simulink model "husky_sim_yichu_MPC_test"  (R2019b)
settings: Solver=ode4  StartTime=0.0  StopTime=5  FixedStep=Ts  MaxStep=0.001  RelTol=1e-3
InitFcn:
  | init_model;
values from neighbouring files (symbols this model uses):
  desired_input = [0,0,0,0,0,0,0,0,0,0,0,0]    [control_params_init.m]
  m = getfield(leg,'mass')    [dynamic_test.m]    (also in pen_init.m = link2.mass; test.mat = 2.2337)
  q_BL_K0 = initial_angle(12)    [func_params_ext.m]
  q_BR_K0 = initial_angle(9)    [func_params_ext.m]
  q_FL_K0 = initial_angle(6)    [func_params_ext.m]
  q_FR_K0 = initial_angle(3)    [func_params_ext.m]
undefined symbols (not defined in the file or in its folder): body, femur_left, femur_right, hip_left, hip_right, hipf_ctrl, hips_ctrl, knee_ctrl, link_left, link_right, tarsus_left, tarsus_right, tibia_left, tibia_right, X, Y, Z
libraries: sm_lib x247, nesl_utility x86, simulink x36, Contact_Forces_Lib x20
(part 1 of 9)
settings Model: PauseTimes=0.4  NumberOfSteps=10  SnapshotBufferSize=100  SnapshotInterval=20  Creator=Yang  LastModifiedBy=yichu
settings SolverCC: AlgebraicLoopSolver=LineSearch  SolverResetMethod=Robust
settings SFSimCC: CustomCodeUndefinedFunction=UseInterfaceOnly
settings RTWCC: Description=Simulink Desktop Real-Time  SystemTargetFile=sldrt.tlc  TemplateMakefile=sldrt.tmf  RTWCompilerOptimization=on
settings CodeAppCC: MaxIdLength=95
settings SimulinkDesktopRealTimeCC: TargetPreCompLibLocation=D:\Program Files\MATLAB\toolbox\sldrt\lib\win64  PreserveStateflowLocalDataDimensions=off
settings DiagnosticsConfigSet: SimMechanicsRigidlyBoundBlock=warning

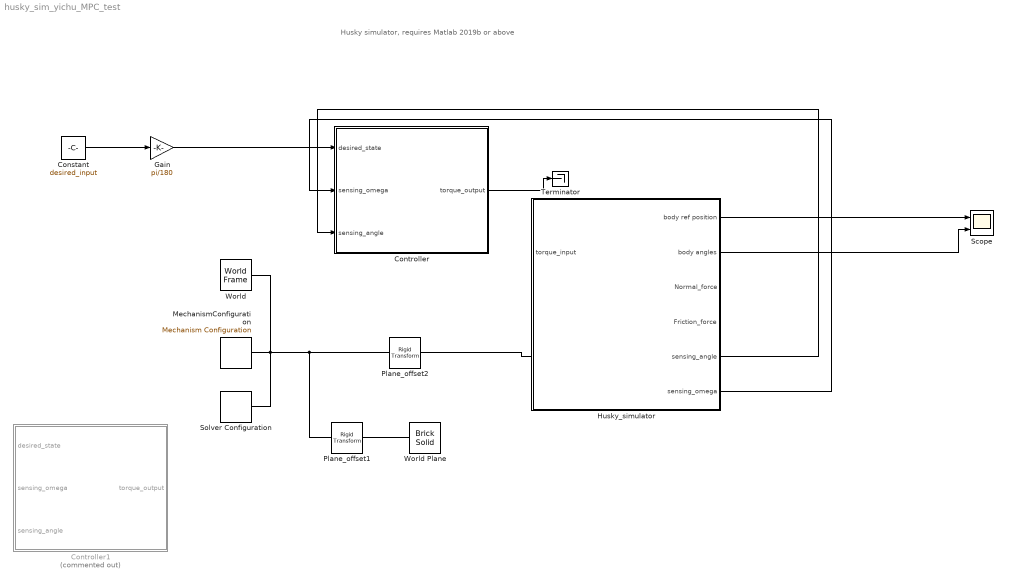
== system husky_sim_yichu_MPC_test ==
  note: Husky simulator, requires Matlab 2019b or above
  Constant : Constant  Value=desired_input
  Controller : Subsystem
  Controller1 : Subsystem  Commented=on
  Gain : Gain  Gain=pi/180
  Husky_simulator : Subsystem
  MechanismConfiguration : sm_lib/Utilities/Mechanism Configuration  UniformGravity=Constant  GravityVector=[0 0 -9.80665]  GravityUnits=m/s^2  LinearizationDelta=0.001
  Plane_offset1 : sm_lib/Frames and Transforms/Rigid Transform  TranslationMethod=Cartesian  TranslationStandardOffset=0  TranslationLengthUnit=m  TranslationStandardAxis=+Z  TranslationCartesianOffset=[0, 0, 0]  TranslationROffset=0  TranslationROffsetUnits=m  TranslationZOffset=0  TranslationZOffsetUnits=m  TranslationThetaOffset=0  TranslationThetaOffsetUnits=deg  RotationMethod=RotationSequence  RotationAngleUnits=deg  RotationStandardAxis=+Z  RotationAngle=0.0  RotationArbitraryAxis=[0 0 1]  FollAlignAxisA=+X  BaseAlignAxisA=+Y  FollAlignAxisB=+Y  BaseAlignAxisB=+Z  RotationSequenceAxes=BaseAxes  RotationSequence=XYZ  RotationSequenceAngles=[0, 0, 0]  RotationSequenceAnglesUnits=rad  RotationMatrix=[1 0 0; 0 1 0; 0 0 1]
  Plane_offset2 : sm_lib/Frames and Transforms/Rigid Transform  TranslationMethod=Cartesian  TranslationStandardOffset=0  TranslationLengthUnit=m  TranslationStandardAxis=+Z  TranslationCartesianOffset=[0, 0, 0]  TranslationROffset=0  TranslationROffsetUnits=m  TranslationZOffset=0  TranslationZOffsetUnits=m  TranslationThetaOffset=0  TranslationThetaOffsetUnits=deg  RotationMethod=StandardAxis  RotationAngleUnits=deg  RotationStandardAxis=+Z  RotationAngle=-90  RotationArbitraryAxis=[0 0 1]  FollAlignAxisA=+X  BaseAlignAxisA=+Y  FollAlignAxisB=+Y  BaseAlignAxisB=+Z  RotationSequenceAxes=BaseAxes  RotationSequence=XYZ  RotationSequenceAngles=[0, 0, 0]  RotationSequenceAnglesUnits=rad  RotationMatrix=[1 0 0; 0 1 0; 0 0 1]
  Scope : Scope  NumInputPorts=2
  Solver Configuration : nesl_utility/Solver Configuration  PhysicalDomain=network_engine_domain  SubClassName=solver  LeftPortType=input  RightPortType=generic  Tones=[]  Harmonics=[]  SimulateNoise=off  Profile=off  UseLocalSampling=off  EnableSwitchedLinearOptims=on  FrequencyDomain=off  UseCCode=off  RelTol=0.001  AbsTol=1e-06  MinStep=1e-09  ToWorkspace=off  RevertToSquareIcSolve=off  NumHomotopyIterations=100  PhasorMode=off  PhasorModeNumHarmonics=1  DoDC=off  ResidualTolerance=1e-09  UseLocalSolver=off  LocalSolverChoice=NE_BACKWARD_EULER_ADVANCER  LocalSolverSampleTime=0.001  DoFixedCost=off  MaxNonlinIter=3  MaxModeIter=2  LinearAlgebra=auto  EquationFormulation=NE_TIME_EF  DelaysMemoryBudget=1024  AutomaticFiltering=on  FilteringTimeConstant=0.001  PartitionStorageMethod=AS_NEEDED  PartitionMemoryBudget=1024  PartitionMethod=ROBUST
  Terminator : Terminator
  World : sm_lib/Frames and Transforms/World Frame
  "World Plane " : sm_lib/Body Elements/Brick Solid  GraphicAmbientColor=[0.15 0.15 0.15 1.0]  BasedOnType=Density  BrickDimensions=[5 5 0.02]  BrickDimensionUnits=m  CenterOfMass=[0 0 0]  CenterOfMassUnits=m  GraphicDiffuseColor=[0.5 0.5 0.5]  Density=1000  DensityUnits=kg/m^3  DoExposeReferenceFrame=on  GraphicEmissiveColor=[0.0 0.0 0.0 1.0]  ExportEntireGeometry=off  SerializedFrames=<Frames/>  MarkerShape=Sphere  MarkerSize=10  GraphicType=FromGeometry  InertiaType=CalculateFromGeometry  Mass=1  MassUnits=kg  MomentsOfInertia=[1 1 1]  MomentsOfInertiaUnits=kg*m^2  GraphicOpacity=1.0  ProductsOfInertia=[0 0 0]  ProductsOfInertiaUnits=kg*m^2  GraphicShininess=75  GraphicSpecularColor=[0.5 0.5 0.5 1.0]  GraphicVisPropType=SimpleVisualProperties
  wires:
  Controller/1(torque_output) -> Terminator/1
  Husky_simulator/5(sensing_angle) -> Controller/3(sensing_angle)
  Husky_simulator/6(sensing_omega) -> Controller/2(sensing_omega)
  Constant/1 -> Gain/1
  Gain/1 -> Controller/1("desired_state ")
  Husky_simulator/2(body angles) -> Scope/2
  Husky_simulator/1(body ref position) -> Scope/1
  connections:
  Plane_offset2/RConn1 -- Husky_simulator/LConn1
  Plane_offset1/RConn1 -- "World Plane "/RConn1
  Plane_offset1/LConn1 -- Plane_offset2/LConn1 -- Solver Configuration/RConn1 -- World/RConn1 -- MechanismConfiguration/RConn1

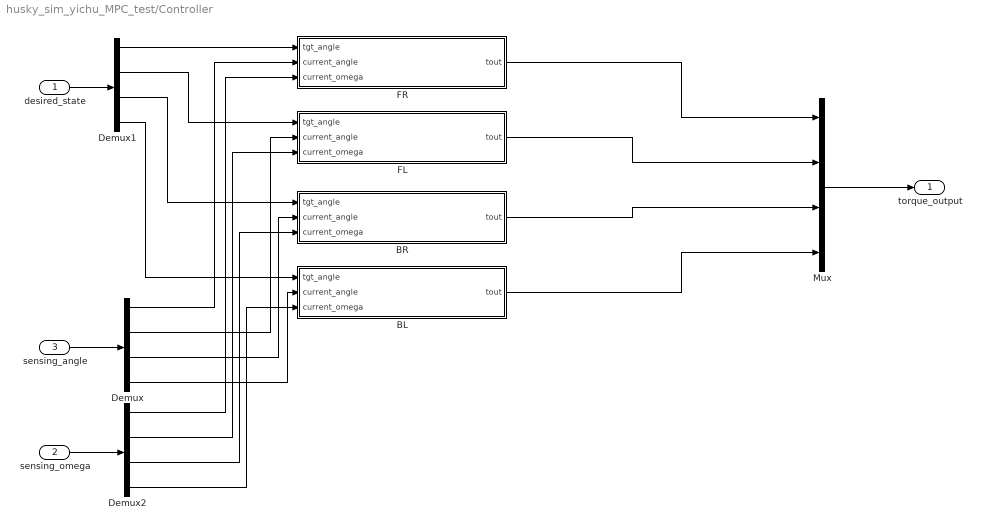
== system husky_sim_yichu_MPC_test/Controller ==
  "desired_state " : Inport
  sensing_omega : Inport  Port=2
  sensing_angle : Inport  Port=3
  BL : Subsystem
  BR : Subsystem
  Demux : Demux
  Demux1 : Demux
  Demux2 : Demux
  FL : Subsystem
  "FR " : Subsystem
  Mux : Mux
  torque_output : Outport
  wires:
  sensing_angle/1 -> Demux/1
  "desired_state "/1 -> Demux1/1
  Demux/1 -> "FR "/2("current_angle ")
  Demux/2 -> FL/2("current_angle ")
  Demux/3 -> BR/2("current_angle ")
  Demux/4 -> BL/2("current_angle ")
  Demux1/1 -> "FR "/1(tgt_angle)
  Demux1/2 -> FL/1(tgt_angle)
  Demux1/3 -> BR/1(tgt_angle)
  Demux1/4 -> BL/1(tgt_angle)
  Demux2/4 -> BL/3(current_omega)
  sensing_omega/1 -> Demux2/1
  Demux2/1 -> "FR "/3(current_omega)
  Demux2/3 -> BR/3(current_omega)
  Demux2/2 -> FL/3(current_omega)
  "FR "/1("tout ") -> Mux/1
  FL/1("tout ") -> Mux/2
  BR/1("tout ") -> Mux/3
  BL/1("tout ") -> Mux/4
  Mux/1 -> torque_output/1

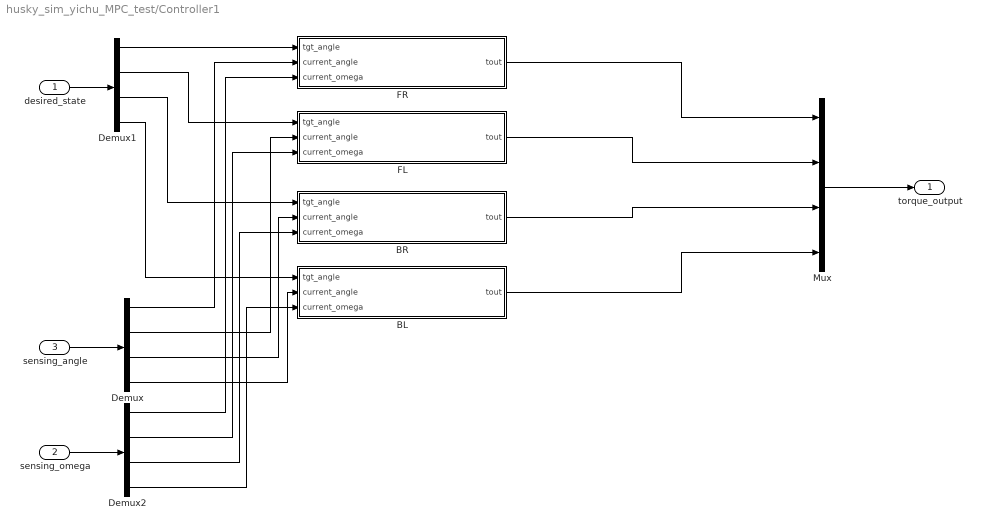
== system husky_sim_yichu_MPC_test/Controller1 ==
  "desired_state " : Inport
  sensing_omega : Inport  Port=2
  sensing_angle : Inport  Port=3
  BL : Subsystem
  BR : Subsystem
  Demux : Demux
  Demux1 : Demux
  Demux2 : Demux
  FL : Subsystem
  "FR " : Subsystem
  Mux : Mux
  torque_output : Outport
  wires:
  sensing_angle/1 -> Demux/1
  "desired_state "/1 -> Demux1/1
  Demux/1 -> "FR "/2("current_angle ")
  Demux/2 -> FL/2("current_angle ")
  Demux/3 -> BR/2("current_angle ")
  Demux/4 -> BL/2("current_angle ")
  Demux1/1 -> "FR "/1(tgt_angle)
  Demux1/2 -> FL/1(tgt_angle)
  Demux1/3 -> BR/1(tgt_angle)
  Demux1/4 -> BL/1(tgt_angle)
  Demux2/4 -> BL/3(current_omega)
  sensing_omega/1 -> Demux2/1
  Demux2/1 -> "FR "/3(current_omega)
  Demux2/3 -> BR/3(current_omega)
  Demux2/2 -> FL/3(current_omega)
  "FR "/1("tout ") -> Mux/1
  FL/1("tout ") -> Mux/2
  BR/1("tout ") -> Mux/3
  BL/1("tout ") -> Mux/4
  Mux/1 -> torque_output/1

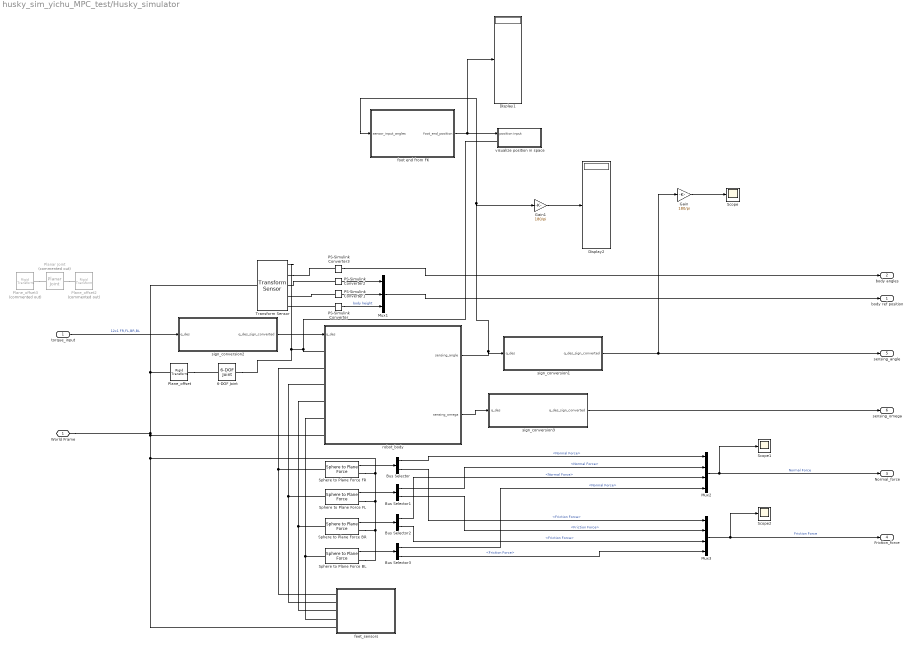
== system husky_sim_yichu_MPC_test/Husky_simulator ==
  "torque_input " : Inport
  6-DOF Joint : sm_lib/Joints/6-DOF Joint  JointMode=Normal  SenseConstraintForce=off  SenseConstraintForceX=off  SenseConstraintForceY=off  SenseConstraintForceZ=off  SenseConstraintTorque=off  SenseConstraintTorqueX=off  SenseConstraintTorqueY=off  SenseConstraintTorqueZ=off  SenseTotalForce=off  SenseTotalForceX=off  SenseTotalForceY=off  SenseTotalForceZ=off  SenseTotalTorque=off  SenseTotalTorqueX=off  SenseTotalTorqueY=off  SenseTotalTorqueZ=off  CompositeWrenchDir=FollowerOnBase  CompositeWrenchFrame=BaseFrame  PxEquilibriumPosition=0  PxEquilibriumPositionUnits=m  PxSpringStiffness=0  PxSpringStiffnessUnits=N/m  PxDampingCoefficient=0  PxDampingCoefficientUnits=N/(m/s)  PxTorqueActuationMode=NoTorque  PxMotionActuationMode=ComputedMotion  PxSensePosition=off  PxSenseVelocity=off  PxSenseAcceleration=off  PxSenseTorqueForce=off  PxSenseLowerLimitTorqueForce=off  PxSenseUpperLimitTorqueForce=off  PxLowerLimitSpecify=off  PxLowerLimitBound=-1  PxLowerLimitBoundUnits=m  PxLowerLimitStiffness=1e6  PxLowerLimitStiffnessUnits=N/m  PxLowerLimitDamping=1e3  PxLowerLimitDampingUnits=N/(m/s)  PxLowerLimitTransitionRegionWidth=1e-4  PxLowerLimitTransitionRegionWidthUnits=m  PxUpperLimitSpecify=off  PxUpperLimitBound=1  PxUpperLimitBoundUnits=m  PxUpperLimitStiffness=1e6  PxUpperLimitStiffnessUnits=N/m  PxUpperLimitDamping=1e3  PxUpperLimitDampingUnits=N/(m/s)  PxUpperLimitTransitionRegionWidth=1e-4  PxUpperLimitTransitionRegionWidthUnits=m  PxPositionTargetSpecify=off  PxPositionTargetPriority=High  PxPositionTargetValue=0  PxPositionTargetValueUnits=m  PxVelocityTargetSpecify=off  PxVelocityTargetPriority=High  PxVelocityTargetValue=0  PxVelocityTargetValueUnits=m/s  PyEquilibriumPosition=0  PyEquilibriumPositionUnits=m  PySpringStiffness=0  PySpringStiffnessUnits=N/m  PyDampingCoefficient=0  PyDampingCoefficientUnits=N/(m/s)  PyTorqueActuationMode=NoTorque  PyMotionActuationMode=ComputedMotion  PySensePosition=off  PySenseVelocity=off  PySenseAcceleration=off  PySenseTorqueForce=off  PySenseLowerLimitTorqueForce=off  PySenseUpperLimitTorqueForce=off  PyLowerLimitSpecify=off  PyLowerLimitBound=-1  PyLowerLimitBoundUnits=m  PyLowerLimitStiffness=1e6  PyLowerLimitStiffnessUnits=N/m  PyLowerLimitDamping=1e3  PyLowerLimitDampingUnits=N/(m/s)  PyLowerLimitTransitionRegionWidth=1e-4  PyLowerLimitTransitionRegionWidthUnits=m  PyUpperLimitSpecify=off  PyUpperLimitBound=1  PyUpperLimitBoundUnits=m  PyUpperLimitStiffness=1e6  PyUpperLimitStiffnessUnits=N/m  PyUpperLimitDamping=1e3  PyUpperLimitDampingUnits=N/(m/s)  PyUpperLimitTransitionRegionWidth=1e-4  PyUpperLimitTransitionRegionWidthUnits=m  PyPositionTargetSpecify=off  PyPositionTargetPriority=High  PyPositionTargetValue=0  PyPositionTargetValueUnits=m  PyVelocityTargetSpecify=off  PyVelocityTargetPriority=High  PyVelocityTargetValue=0  PyVelocityTargetValueUnits=m/s  PzEquilibriumPosition=0  PzEquilibriumPositionUnits=m  PzSpringStiffness=0  PzSpringStiffnessUnits=N/m  PzDampingCoefficient=0  PzDampingCoefficientUnits=N/(m/s)  PzTorqueActuationMode=NoTorque  PzMotionActuationMode=ComputedMotion  PzSensePosition=off  PzSenseVelocity=off  PzSenseAcceleration=off  PzSenseTorqueForce=off  PzSenseLowerLimitTorqueForce=off  PzSenseUpperLimitTorqueForce=off  PzLowerLimitSpecify=off  PzLowerLimitBound=-1  PzLowerLimitBoundUnits=m  PzLowerLimitStiffness=1e6  PzLowerLimitStiffnessUnits=N/m  PzLowerLimitDamping=1e3  PzLowerLimitDampingUnits=N/(m/s)  PzLowerLimitTransitionRegionWidth=1e-4  PzLowerLimitTransitionRegionWidthUnits=m  PzUpperLimitSpecify=off  PzUpperLimitBound=1  PzUpperLimitBoundUnits=m  PzUpperLimitStiffness=1e6  PzUpperLimitStiffnessUnits=N/m  PzUpperLimitDamping=1e3  PzUpperLimitDampingUnits=N/(m/s)  PzUpperLimitTransitionRegionWidth=1e-4  PzUpperLimitTransitionRegionWidthUnits=m  PzPositionTargetSpecify=off  PzPositionTargetPriority=High  PzPositionTargetValue=0  PzPositionTargetValueUnits=m  PzVelocityTargetSpecify=off  PzVelocityTargetPriority=High  PzVelocityTargetValue=0  PzVelocityTargetValueUnits=m/s  SphDefPosRotationMethod=None  SphDefPosRotationAngleUnits=deg  SphDefPosRotationStandardAxis=+Z  SphDefPosRotationAngle=0.0  SphDefPosRotationArbitraryAxis=[0 0 1]  SphDefPosFollAlignAxisA=+X  SphDefPosBaseAlignAxisA=+Y  SphDefPosFollAlignAxisB=+Y  SphDefPosBaseAlignAxisB=+Z  SphDefPosRotationSequenceAxes=FollowerAxes  SphDefPosRotationSequence=XYX  SphDefPosRotationSequenceAngles=[0 0 0]  SphDefPosRotationSequenceAnglesUnits=deg  SphDefPosRotationMatrix=[1 0 0; 0 1 0; 0 0 1]  SphEqPosRotationMethod=None  SphEqPosRotationAngleUnits=deg  SphEqPosRotationStandardAxis=+Z  SphEqPosRotationAngle=0.0  SphEqPosRotationArbitraryAxis=[0 0 1]  SphEqPosFollAlignAxisA=+X  SphEqPosBaseAlignAxisA=+Y  SphEqPosFollAlignAxisB=+Y  SphEqPosBaseAlignAxisB=+Z  SphEqPosRotationSequenceAxes=FollowerAxes  SphEqPosRotationSequence=XYX  SphEqPosRotationSequenceAngles=[0 0 0]  SphEqPosRotationSequenceAnglesUnits=deg  SphEqPosRotationMatrix=[1 0 0; 0 1 0; 0 0 1]  SphSpringStiffness=0  SphSpringStiffnessUnits=N*m/deg  SphDampingCoefficient=0  SphDampingCoefficientUnits=N*m/(deg/s)  SphActuateTorqueX=off  SphActuateTorqueY=off  SphActuateTorqueZ=off  SphActuateTorque=off  SphTorqueActuationMode=NoTorque  SphMotionActuationMode=ComputedMotion  SphActuationFrame=BaseFrame  SphSensePosition=off  SphSenseVelocityX=off  SphSenseVelocityY=off  SphSenseVelocityZ=off  SphSenseVelocity=off  SphSenseAccelerationX=off  SphSenseAccelerationY=off  SphSenseAccelerationZ=off  SphSenseAcceleration=off  SphSenseTorqueX=off  SphSenseTorqueY=off  SphSenseTorqueZ=off  SphSenseTorqueForce=off  SphSenseLowerLimitTorqueMag=off  SphSenseUpperLimitTorqueMag=off  SphSensingFrame=BaseFrame  SphLowerLimitSpecify=off  SphLowerLimitBound=15  SphLowerLimitBoundUnits=deg  SphLowerLimitStiffness=1e4  SphLowerLimitStiffnessUnits=N*m/deg  SphLowerLimitDamping=10  SphLowerLimitDampingUnits=N*m/(deg/s)  SphLowerLimitTransitionRegionWidth=0.1  SphLowerLimitTransitionRegionWidthUnits=deg  SphUpperLimitSpecify=off  SphUpperLimitBound=45  SphUpperLimitBoundUnits=deg  SphUpperLimitStiffness=1e4  SphUpperLimitStiffnessUnits=N*m/deg  SphUpperLimitDamping=10  SphUpperLimitDampingUnits=N*m/(deg/s)  SphUpperLimitTransitionRegionWidth=0.1  SphUpperLimitTransitionRegionWidthUnits=deg  SphPositionTargetRotationMethod=None  SphPositionTargetRotationAngleUnits=deg  SphPositionTargetRotationStandardAxis=+Z  SphPositionTargetRotationAngle=0.0  SphPositionTargetRotationArbitraryAxis=[0 0 1]  SphPositionTargetFollAlignAxisA=+X  SphPositionTargetBaseAlignAxisA=+Y  SphPositionTargetFollAlignAxisB=+Y  SphPositionTargetBaseAlignAxisB=+Z  SphPositionTargetRotationSequenceAxes=FollowerAxes  SphPositionTargetRotationSequence=XYX  SphPositionTargetRotationSequenceAngles=[0 0 0]  SphPositionTargetRotationSequenceAnglesUnits=deg  SphPositionTargetRotationMatrix=[1 0 0; 0 1 0; 0 0 1]  SphPositionTargetSpecify=off  SphPositionTargetPriority=High  SphVelocityTargetValue=[0 0 0]  SphVelocityTargetValueUnits=deg/s  SphVelocityTargetSpecify=off  SphVelocityTargetPriority=High  SphVelocityTargetInFollowerFrame=on
  Bus Selector{,1..3} (4 alike) : BusSelector  OutputSignals=Normal Force,Friction Force
  Display1 : Display
  Display2 : Display
  Gain : Gain  Gain=180/pi
  Gain1 : Gain  Gain=180/pi
  Mux1 : Mux  Inputs=3
  Mux2 : Mux
  Mux3 : Mux
  PS-Simulink Converter{,1..3} (4 alike) : nesl_utility/PS-Simulink Converter  PhysicalDomain=network_engine_domain  SubClassName=ps_output  LeftPortType=input  RightPortType=output  PseudoPeriodic=off  Frequencies=[]  Unit=inherit  AffineConversion=off
  Planar Joint : sm_lib/Joints/Planar Joint  Commented=on  JointMode=Normal  SenseConstraintForce=off  SenseConstraintForceX=off  SenseConstraintForceY=off  SenseConstraintForceZ=off  SenseConstraintTorque=off  SenseConstraintTorqueX=off  SenseConstraintTorqueY=off  SenseConstraintTorqueZ=off  SenseTotalForce=off  SenseTotalForceX=off  SenseTotalForceY=off  SenseTotalForceZ=off  SenseTotalTorque=off  SenseTotalTorqueX=off  SenseTotalTorqueY=off  SenseTotalTorqueZ=off  CompositeWrenchDir=FollowerOnBase  CompositeWrenchFrame=BaseFrame  PxEquilibriumPosition=0  PxEquilibriumPositionUnits=m  PxSpringStiffness=0  PxSpringStiffnessUnits=N/m  PxDampingCoefficient=0  PxDampingCoefficientUnits=N/(m/s)  PxTorqueActuationMode=NoTorque  PxMotionActuationMode=ComputedMotion  PxSensePosition=off  PxSenseVelocity=off  PxSenseAcceleration=off  PxSenseTorqueForce=off  PxSenseLowerLimitTorqueForce=off  PxSenseUpperLimitTorqueForce=off  PxLowerLimitSpecify=off  PxLowerLimitBound=-1  PxLowerLimitBoundUnits=m  PxLowerLimitStiffness=1e6  PxLowerLimitStiffnessUnits=N/m  PxLowerLimitDamping=1e3  PxLowerLimitDampingUnits=N/(m/s)  PxLowerLimitTransitionRegionWidth=1e-4  PxLowerLimitTransitionRegionWidthUnits=m  PxUpperLimitSpecify=off  PxUpperLimitBound=1  PxUpperLimitBoundUnits=m  PxUpperLimitStiffness=1e6  PxUpperLimitStiffnessUnits=N/m  PxUpperLimitDamping=1e3  PxUpperLimitDampingUnits=N/(m/s)  PxUpperLimitTransitionRegionWidth=1e-4  PxUpperLimitTransitionRegionWidthUnits=m  PxPositionTargetSpecify=off  PxPositionTargetPriority=High  PxPositionTargetValue=0  PxPositionTargetValueUnits=m  PxVelocityTargetSpecify=off  PxVelocityTargetPriority=High  PxVelocityTargetValue=0  PxVelocityTargetValueUnits=m/s  PyEquilibriumPosition=0  PyEquilibriumPositionUnits=m  PySpringStiffness=0  PySpringStiffnessUnits=N/m  PyDampingCoefficient=0  PyDampingCoefficientUnits=N/(m/s)  PyTorqueActuationMode=NoTorque  PyMotionActuationMode=ComputedMotion  PySensePosition=off  PySenseVelocity=off  PySenseAcceleration=off  PySenseTorqueForce=off  PySenseLowerLimitTorqueForce=off  PySenseUpperLimitTorqueForce=off  PyLowerLimitSpecify=off  PyLowerLimitBound=-1  PyLowerLimitBoundUnits=m  PyLowerLimitStiffness=1e6  PyLowerLimitStiffnessUnits=N/m  PyLowerLimitDamping=1e3  PyLowerLimitDampingUnits=N/(m/s)  PyLowerLimitTransitionRegionWidth=1e-4  PyLowerLimitTransitionRegionWidthUnits=m  PyUpperLimitSpecify=off  PyUpperLimitBound=1  PyUpperLimitBoundUnits=m  PyUpperLimitStiffness=1e6  PyUpperLimitStiffnessUnits=N/m  PyUpperLimitDamping=1e3  PyUpperLimitDampingUnits=N/(m/s)  PyUpperLimitTransitionRegionWidth=1e-4  PyUpperLimitTransitionRegionWidthUnits=m  PyPositionTargetSpecify=off  PyPositionTargetPriority=High  PyPositionTargetValue=0  PyPositionTargetValueUnits=m  PyVelocityTargetSpecify=off  PyVelocityTargetPriority=High  PyVelocityTargetValue=0  PyVelocityTargetValueUnits=m/s  RzEquilibriumPosition=0  RzEquilibriumPositionUnits=deg  RzSpringStiffness=0  RzSpringStiffnessUnits=N*m/deg  RzDampingCoefficient=0  RzDampingCoefficientUnits=N*m/(deg/s)  RzTorqueActuationMode=NoTorque  RzMotionActuationMode=ComputedMotion  RzSensePosition=off  RzSenseVelocity=off  RzSenseAcceleration=off  RzSenseTorqueForce=off  RzSenseLowerLimitTorqueForce=off  RzSenseUpperLimitTorqueForce=off  RzLowerLimitSpecify=off  RzLowerLimitBound=-90  RzLowerLimitBoundUnits=deg  RzLowerLimitStiffness=1e4  RzLowerLimitStiffnessUnits=N*m/deg  RzLowerLimitDamping=10  RzLowerLimitDampingUnits=N*m/(deg/s)  RzLowerLimitTransitionRegionWidth=0.1  RzLowerLimitTransitionRegionWidthUnits=deg  RzUpperLimitSpecify=off  RzUpperLimitBound=90  RzUpperLimitBoundUnits=deg  RzUpperLimitStiffness=1e4  RzUpperLimitStiffnessUnits=N*m/deg  RzUpperLimitDamping=10  RzUpperLimitDampingUnits=N*m/(deg/s)  RzUpperLimitTransitionRegionWidth=0.1  RzUpperLimitTransitionRegionWidthUnits=deg  RzPositionTargetSpecify=off  RzPositionTargetPriority=High  RzPositionTargetValue=0  RzPositionTargetValueUnits=deg  RzVelocityTargetSpecify=off  RzVelocityTargetPriority=High  RzVelocityTargetValue=0  RzVelocityTargetValueUnits=deg/s
  Plane_offset : sm_lib/Frames and Transforms/Rigid Transform  TranslationMethod=Cartesian  TranslationStandardOffset=0  TranslationLengthUnit=m  TranslationStandardAxis=+Z  TranslationCartesianOffset=p_b0  TranslationROffset=0  TranslationROffsetUnits=m  TranslationZOffset=0  TranslationZOffsetUnits=m  TranslationThetaOffset=0  TranslationThetaOffsetUnits=deg  RotationMethod=RotationSequence  RotationAngleUnits=deg  RotationStandardAxis=+Z  RotationAngle=0.0  RotationArbitraryAxis=[0 0 1]  FollAlignAxisA=+X  BaseAlignAxisA=+Y  FollAlignAxisB=+Y  BaseAlignAxisB=+Z  RotationSequenceAxes=BaseAxes  RotationSequence=XYZ  RotationSequenceAngles=[0, 0, 0]  RotationSequenceAnglesUnits=deg  RotationMatrix=[1 0 0; 0 1 0; 0 0 1]
  Plane_offset2 : sm_lib/Frames and Transforms/Rigid Transform  Commented=on  TranslationMethod=Cartesian  TranslationStandardOffset=0  TranslationLengthUnit=m  TranslationStandardAxis=+Z  TranslationCartesianOffset=[0, 0, 0]  TranslationROffset=0  TranslationROffsetUnits=m  TranslationZOffset=0  TranslationZOffsetUnits=m  TranslationThetaOffset=0  TranslationThetaOffsetUnits=deg  RotationMethod=RotationSequence  RotationAngleUnits=deg  RotationStandardAxis=+Z  RotationAngle=0.0  RotationArbitraryAxis=[0 0 1]  FollAlignAxisA=+X  BaseAlignAxisA=+Y  FollAlignAxisB=+Y  BaseAlignAxisB=+Z  RotationSequenceAxes=BaseAxes  RotationSequence=XYZ  RotationSequenceAngles=[-90, 0, 0]  RotationSequenceAnglesUnits=deg  RotationMatrix=[1 0 0; 0 1 0; 0 0 1]
  Plane_offset3 : sm_lib/Frames and Transforms/Rigid Transform  Commented=on  TranslationMethod=Cartesian  TranslationStandardOffset=0  TranslationLengthUnit=m  TranslationStandardAxis=+Z  TranslationCartesianOffset=[0, 0, 0]  TranslationROffset=0  TranslationROffsetUnits=m  TranslationZOffset=0  TranslationZOffsetUnits=m  TranslationThetaOffset=0  TranslationThetaOffsetUnits=deg  RotationMethod=RotationSequence  RotationAngleUnits=deg  RotationStandardAxis=+Z  RotationAngle=0.0  RotationArbitraryAxis=[0 0 1]  FollAlignAxisA=+X  BaseAlignAxisA=+Y  FollAlignAxisB=+Y  BaseAlignAxisB=+Z  RotationSequenceAxes=BaseAxes  RotationSequence=XYZ  RotationSequenceAngles=[90, 0, 0]  RotationSequenceAnglesUnits=deg  RotationMatrix=[1 0 0; 0 1 0; 0 0 1]
  Scope : Scope
  Scope1 : Scope
  Scope2 : Scope
  "Sphere to Plane Force BL " : Contact_Forces_Lib/3D/Sphere to Plane Force  sphere_rad=0.021  plane_lenx=5  plane_leny=5  plane_depth=0.01  force_law=Linear  k_contact=c_k  b_contact=c_b  pen_full_damp_F=1e-4  pen_exponent=1  custom_param_1=1  custom_param_2=1  friction_law=Stick-Slip Continuous  mu_kinetic=mu_k  mu_static=mu_s  v_thr=v_th  vis_on=off  vis_opc_en=0  vis_len_plaBz=0.001  vis_clr=[0.9 0.2 0.2]  vis_opc=0.7
  "Sphere to Plane Force BR " : Contact_Forces_Lib/3D/Sphere to Plane Force  sphere_rad=0.021  plane_lenx=5  plane_leny=5  plane_depth=0.01  force_law=Linear  k_contact=c_k  b_contact=c_b  pen_full_damp_F=1e-4  pen_exponent=1  custom_param_1=1  custom_param_2=1  friction_law=Stick-Slip Continuous  mu_kinetic=mu_k  mu_static=mu_s  v_thr=v_th  vis_on=off  vis_opc_en=0  vis_len_plaBz=0.001  vis_clr=[0.9 0.2 0.2]  vis_opc=0.7
  Sphere to Plane Force FL : Contact_Forces_Lib/3D/Sphere to Plane Force  sphere_rad=0.021  plane_lenx=5  plane_leny=5  plane_depth=0.01  force_law=Linear  k_contact=c_k  b_contact=c_b  pen_full_damp_F=1e-4  pen_exponent=1  custom_param_1=1  custom_param_2=1  friction_law=Stick-Slip Continuous  mu_kinetic=mu_k  mu_static=mu_s  v_thr=v_th  vis_on=off  vis_opc_en=0  vis_len_plaBz=0.001  vis_clr=[0.9 0.2 0.2]  vis_opc=0.7
  Sphere to Plane Force FR : Contact_Forces_Lib/3D/Sphere to Plane Force  sphere_rad=0.021  plane_lenx=5  plane_leny=5  plane_depth=0.01  force_law=Linear  k_contact=c_k  b_contact=c_b  pen_full_damp_F=1e-4  pen_exponent=1  custom_param_1=1  custom_param_2=1  friction_law=Stick-Slip Continuous  mu_kinetic=mu_k  mu_static=mu_s  v_thr=v_th  vis_on=off  vis_opc_en=0  vis_len_plaBz=0.001  vis_clr=[0.9 0.2 0.2]  vis_opc=0.7
  Transform Sensor : sm_lib/Frames and Transforms/Transform Sensor  MeasurementFrame=World  SenseAngle=off  SenseAxis=off  SenseAngle1=off  SenseAngle2=off  SenseAngle3=off  SenseQ=on  SenseR=off  SenseOmegaX=off  SenseOmegaY=off  SenseOmegaZ=off  SenseOmega1=off  SenseOmega2=off  SenseOmega3=off  SenseQDot=off  SenseRDot=off  SenseAlphaX=off  SenseAlphaY=off  SenseAlphaZ=off  SenseAlpha1=off  SenseAlpha2=off  SenseAlpha3=off  SenseQDDot=off  SenseRDDot=off  SenseX=on  SenseY=on  SenseZ=on  SenseRad=off  SenseAzim=off  SenseDist=off  SenseInc=off  SenseXDot=off  SenseYDot=off  SenseZDot=off  SenseRadDot=off  SenseAzimDot=off  SenseDistDot=off  SenseIncDot=off  SenseXDDot=off  SenseYDDot=off  SenseZDDot=off  SenseRadDDot=off  SenseAzimDDot=off  SenseDistDDot=off  SenseIncDDot=off
  feet_sensors : Subsystem
  "foot end from FK " : Subsystem
  robot_body : Subsystem
  sign_conversion1 : MATLAB Function  TreatAsAtomicUnit=on
  sign_conversion2 : MATLAB Function  TreatAsAtomicUnit=on
  sign_conversion3 : MATLAB Function  TreatAsAtomicUnit=on
  "visualize position in space " : Subsystem
  World Frame : PMIOPort  Side=Left
  body ref position : Outport
  body angles : Outport  Port=2
  Normal_force : Outport  Port=3
  Friction_force : Outport  Port=4
  sensing_angle : Outport  Port=5  VectorParamsAs1DForOutWhenUnconnected=off
  sensing_omega : Outport  Port=6  VectorParamsAs1DForOutWhenUnconnected=off
  wires:
  Sphere to Plane Force FR/1 -> Bus Selector/1
  Sphere to Plane Force FL/1 -> Bus Selector1/1
  "Sphere to Plane Force BR "/1 -> Bus Selector2/1
  "Sphere to Plane Force BL "/1 -> Bus Selector3/1
  PS-Simulink Converter/1 -> Mux1/3  "body height"
  PS-Simulink Converter2/1 -> Mux1/1
  PS-Simulink Converter1/1 -> Mux1/2
  Mux1/1 -> body ref position/1
  Mux2/1 -> Scope1/1, Normal_force/1  "Normal Force"
  Mux3/1 -> Friction_force/1, Scope2/1  "Friction Force"
  Bus Selector/1 -> Mux2/1  "<Normal Force>"
  Bus Selector1/1 -> Mux2/2  "<Normal Force>"
  Bus Selector2/1 -> Mux2/3  "<Normal Force>"
  Bus Selector3/1 -> Mux2/4  "<Normal Force>"
  Bus Selector/2 -> Mux3/1  "<Friction Force>"
  Bus Selector1/2 -> Mux3/2  "<Friction Force>"
  Bus Selector2/2 -> Mux3/3  "<Friction Force>"
  Bus Selector3/2 -> Mux3/4  "<Friction Force>"
  PS-Simulink Converter3/1 -> body angles/1
  robot_body/1(sensing_angle) -> "foot end from FK "/1(sensor_input_angles), Gain1/1, sign_conversion1/1(q_des)
  "torque_input "/1 -> sign_conversion2/1(q_des)  "12x1 FR,FL,BR,BL"
  robot_body/2(sensing_omega) -> sign_conversion3/1(q_des)
  Gain/1 -> Scope/1
  sign_conversion3/1(q_des_sign_converted) -> sensing_omega/1
  sign_conversion2/1(q_des_sign_converted) -> robot_body/1(q_des)
  "foot end from FK "/1("foot_end_position ") -> Display1/1, "visualize position in space "/1(position input)
  sign_conversion1/1(q_des_sign_converted) -> Gain/1, sensing_angle/1
  Gain1/1 -> Display2/1
  connections:
  "Sphere to Plane Force BR "/LConn1 -- robot_body/LConn4 -- feet_sensors/LConn3
  "Sphere to Plane Force BL "/LConn1 -- robot_body/LConn5 -- feet_sensors/LConn4
  Sphere to Plane Force FR/LConn1 -- feet_sensors/LConn1 -- robot_body/LConn2
  Sphere to Plane Force FL/LConn1 -- robot_body/LConn3 -- feet_sensors/LConn2
  PS-Simulink Converter/LConn1 -- Transform Sensor/RConn5
  PS-Simulink Converter1/LConn1 -- Transform Sensor/RConn4
  PS-Simulink Converter2/LConn1 -- Transform Sensor/RConn3
  Transform Sensor/RConn2 -- PS-Simulink Converter3/LConn1
  Transform Sensor/LConn1 -- Plane_offset/LConn1 -- robot_body/LConn6 -- feet_sensors/LConn5 -- "Sphere to Plane Force BL "/RConn1 -- "Sphere to Plane Force BR "/RConn1 -- Sphere to Plane Force FL/RConn1 -- Sphere to Plane Force FR/RConn1 -- World Frame/RConn1
  Plane_offset3/RConn1 -- Planar Joint/LConn1
  Planar Joint/RConn1 -- Plane_offset2/LConn1
  Transform Sensor/RConn1 -- 6-DOF Joint/RConn1 -- "visualize position in space "/LConn1 -- robot_body/LConn1
  Plane_offset/RConn1 -- 6-DOF Joint/LConn1

== system husky_sim_yichu_MPC_test/Controller/BL ==
  tgt_angle : Inport
  "current_angle " : Inport  Port=2
  current_omega : Inport  Port=3
  Demux : Demux  Outputs=3
  Demux1 : Demux  Outputs=3
  Demux2 : Demux  Outputs=3
  Mux : Mux  Inputs=3
  "s_joint_ctrl_hip " : Subsystem
  s_joint_ctrl_hip2 : Subsystem
  s_joint_ctrl_knee : Subsystem
  "tout " : Outport
  wires:
  tgt_angle/1 -> Demux/1
  Demux/1 -> "s_joint_ctrl_hip "/1(tgt_angle)
  Demux/2 -> s_joint_ctrl_hip2/1(tgt_angle)
  Demux/3 -> s_joint_ctrl_knee/1(tgt_angle)
  "current_angle "/1 -> Demux1/1
  Demux1/1 -> "s_joint_ctrl_hip "/2("current_angle ")
  Demux1/2 -> s_joint_ctrl_hip2/2("current_angle ")
  Demux1/3 -> s_joint_ctrl_knee/2("current_angle ")
  current_omega/1 -> Demux2/1
  Demux2/1 -> "s_joint_ctrl_hip "/3(current_omega)
  Demux2/2 -> s_joint_ctrl_hip2/3(current_omega)
  Demux2/3 -> s_joint_ctrl_knee/3(current_omega)
  "s_joint_ctrl_hip "/1(tout) -> Mux/1
  s_joint_ctrl_hip2/1(tout) -> Mux/2
  s_joint_ctrl_knee/1(tout) -> Mux/3
  Mux/1 -> "tout "/1

== system husky_sim_yichu_MPC_test/Controller/BR ==
  tgt_angle : Inport
  "current_angle " : Inport  Port=2
  current_omega : Inport  Port=3
  Demux : Demux  Outputs=3
  Demux1 : Demux  Outputs=3
  Demux2 : Demux  Outputs=3
  Mux : Mux  Inputs=3
  "s_joint_ctrl_hip " : Subsystem
  s_joint_ctrl_hip2 : Subsystem
  s_joint_ctrl_knee : Subsystem
  "tout " : Outport
  wires:
  tgt_angle/1 -> Demux/1
  Demux/1 -> "s_joint_ctrl_hip "/1(tgt_angle)
  Demux/2 -> s_joint_ctrl_hip2/1(tgt_angle)
  Demux/3 -> s_joint_ctrl_knee/1(tgt_angle)
  "current_angle "/1 -> Demux1/1
  Demux1/1 -> "s_joint_ctrl_hip "/2("current_angle ")
  Demux1/2 -> s_joint_ctrl_hip2/2("current_angle ")
  Demux1/3 -> s_joint_ctrl_knee/2("current_angle ")
  current_omega/1 -> Demux2/1
  Demux2/1 -> "s_joint_ctrl_hip "/3(current_omega)
  Demux2/2 -> s_joint_ctrl_hip2/3(current_omega)
  Demux2/3 -> s_joint_ctrl_knee/3(current_omega)
  "s_joint_ctrl_hip "/1(tout) -> Mux/1
  s_joint_ctrl_hip2/1(tout) -> Mux/2
  s_joint_ctrl_knee/1(tout) -> Mux/3
  Mux/1 -> "tout "/1

== system husky_sim_yichu_MPC_test/Controller/FL ==
  tgt_angle : Inport
  "current_angle " : Inport  Port=2
  current_omega : Inport  Port=3
  Demux : Demux  Outputs=3
  Demux1 : Demux  Outputs=3
  Demux2 : Demux  Outputs=3
  Mux : Mux  Inputs=3
  "s_joint_ctrl_hip " : Subsystem
  s_joint_ctrl_hip2 : Subsystem
  s_joint_ctrl_knee : Subsystem
  "tout " : Outport
  wires:
  tgt_angle/1 -> Demux/1
  Demux/1 -> "s_joint_ctrl_hip "/1(tgt_angle)
  Demux/2 -> s_joint_ctrl_hip2/1(tgt_angle)
  Demux/3 -> s_joint_ctrl_knee/1(tgt_angle)
  "current_angle "/1 -> Demux1/1
  Demux1/1 -> "s_joint_ctrl_hip "/2("current_angle ")
  Demux1/2 -> s_joint_ctrl_hip2/2("current_angle ")
  Demux1/3 -> s_joint_ctrl_knee/2("current_angle ")
  current_omega/1 -> Demux2/1
  Demux2/1 -> "s_joint_ctrl_hip "/3(current_omega)
  Demux2/2 -> s_joint_ctrl_hip2/3(current_omega)
  Demux2/3 -> s_joint_ctrl_knee/3(current_omega)
  "s_joint_ctrl_hip "/1(tout) -> Mux/1
  s_joint_ctrl_hip2/1(tout) -> Mux/2
  s_joint_ctrl_knee/1(tout) -> Mux/3
  Mux/1 -> "tout "/1

== system husky_sim_yichu_MPC_test/Controller/FR  ==
  tgt_angle : Inport
  "current_angle " : Inport  Port=2
  current_omega : Inport  Port=3
  Demux : Demux  Outputs=3
  Demux1 : Demux  Outputs=3
  Demux2 : Demux  Outputs=3
  Mux : Mux  Inputs=3
  "s_joint_ctrl_hip " : Subsystem
  s_joint_ctrl_hip2 : Subsystem
  s_joint_ctrl_knee : Subsystem
  "tout " : Outport
  wires:
  tgt_angle/1 -> Demux/1
  Demux/1 -> "s_joint_ctrl_hip "/1(tgt_angle)
  Demux/2 -> s_joint_ctrl_hip2/1(tgt_angle)
  Demux/3 -> s_joint_ctrl_knee/1(tgt_angle)
  "current_angle "/1 -> Demux1/1
  Demux1/1 -> "s_joint_ctrl_hip "/2("current_angle ")
  Demux1/2 -> s_joint_ctrl_hip2/2("current_angle ")
  Demux1/3 -> s_joint_ctrl_knee/2("current_angle ")
  current_omega/1 -> Demux2/1
  Demux2/1 -> "s_joint_ctrl_hip "/3(current_omega)
  Demux2/2 -> s_joint_ctrl_hip2/3(current_omega)
  Demux2/3 -> s_joint_ctrl_knee/3(current_omega)
  "s_joint_ctrl_hip "/1(tout) -> Mux/1
  s_joint_ctrl_hip2/1(tout) -> Mux/2
  s_joint_ctrl_knee/1(tout) -> Mux/3
  Mux/1 -> "tout "/1

== system husky_sim_yichu_MPC_test/Controller1/BL ==
  tgt_angle : Inport
  "current_angle " : Inport  Port=2
  current_omega : Inport  Port=3
  Demux : Demux  Outputs=3
  Demux1 : Demux  Outputs=3
  Demux2 : Demux  Outputs=3
  Mux : Mux  Inputs=3
  "s_joint_ctrl_hip " : Subsystem
  s_joint_ctrl_hip2 : Subsystem
  s_joint_ctrl_knee : Subsystem
  "tout " : Outport
  wires:
  tgt_angle/1 -> Demux/1
  Demux/1 -> "s_joint_ctrl_hip "/1(tgt_angle)
  Demux/2 -> s_joint_ctrl_hip2/1(tgt_angle)
  Demux/3 -> s_joint_ctrl_knee/1(tgt_angle)
  "current_angle "/1 -> Demux1/1
  Demux1/1 -> "s_joint_ctrl_hip "/2("current_angle ")
  Demux1/2 -> s_joint_ctrl_hip2/2("current_angle ")
  Demux1/3 -> s_joint_ctrl_knee/2("current_angle ")
  current_omega/1 -> Demux2/1
  Demux2/1 -> "s_joint_ctrl_hip "/3(current_omega)
  Demux2/2 -> s_joint_ctrl_hip2/3(current_omega)
  Demux2/3 -> s_joint_ctrl_knee/3(current_omega)
  "s_joint_ctrl_hip "/1(tout) -> Mux/1
  s_joint_ctrl_hip2/1(tout) -> Mux/2
  s_joint_ctrl_knee/1(tout) -> Mux/3
  Mux/1 -> "tout "/1

== system husky_sim_yichu_MPC_test/Controller1/BR ==
  tgt_angle : Inport
  "current_angle " : Inport  Port=2
  current_omega : Inport  Port=3
  Demux : Demux  Outputs=3
  Demux1 : Demux  Outputs=3
  Demux2 : Demux  Outputs=3
  Mux : Mux  Inputs=3
  "s_joint_ctrl_hip " : Subsystem
  s_joint_ctrl_hip2 : Subsystem
  s_joint_ctrl_knee : Subsystem
  "tout " : Outport
  wires:
  tgt_angle/1 -> Demux/1
  Demux/1 -> "s_joint_ctrl_hip "/1(tgt_angle)
  Demux/2 -> s_joint_ctrl_hip2/1(tgt_angle)
  Demux/3 -> s_joint_ctrl_knee/1(tgt_angle)
  "current_angle "/1 -> Demux1/1
  Demux1/1 -> "s_joint_ctrl_hip "/2("current_angle ")
  Demux1/2 -> s_joint_ctrl_hip2/2("current_angle ")
  Demux1/3 -> s_joint_ctrl_knee/2("current_angle ")
  current_omega/1 -> Demux2/1
  Demux2/1 -> "s_joint_ctrl_hip "/3(current_omega)
  Demux2/2 -> s_joint_ctrl_hip2/3(current_omega)
  Demux2/3 -> s_joint_ctrl_knee/3(current_omega)
  "s_joint_ctrl_hip "/1(tout) -> Mux/1
  s_joint_ctrl_hip2/1(tout) -> Mux/2
  s_joint_ctrl_knee/1(tout) -> Mux/3
  Mux/1 -> "tout "/1

== system husky_sim_yichu_MPC_test/Controller1/FL ==
  tgt_angle : Inport
  "current_angle " : Inport  Port=2
  current_omega : Inport  Port=3
  Demux : Demux  Outputs=3
  Demux1 : Demux  Outputs=3
  Demux2 : Demux  Outputs=3
  Mux : Mux  Inputs=3
  "s_joint_ctrl_hip " : Subsystem
  s_joint_ctrl_hip2 : Subsystem
  s_joint_ctrl_knee : Subsystem
  "tout " : Outport
  wires:
  tgt_angle/1 -> Demux/1
  Demux/1 -> "s_joint_ctrl_hip "/1(tgt_angle)
  Demux/2 -> s_joint_ctrl_hip2/1(tgt_angle)
  Demux/3 -> s_joint_ctrl_knee/1(tgt_angle)
  "current_angle "/1 -> Demux1/1
  Demux1/1 -> "s_joint_ctrl_hip "/2("current_angle ")
  Demux1/2 -> s_joint_ctrl_hip2/2("current_angle ")
  Demux1/3 -> s_joint_ctrl_knee/2("current_angle ")
  current_omega/1 -> Demux2/1
  Demux2/1 -> "s_joint_ctrl_hip "/3(current_omega)
  Demux2/2 -> s_joint_ctrl_hip2/3(current_omega)
  Demux2/3 -> s_joint_ctrl_knee/3(current_omega)
  "s_joint_ctrl_hip "/1(tout) -> Mux/1
  s_joint_ctrl_hip2/1(tout) -> Mux/2
  s_joint_ctrl_knee/1(tout) -> Mux/3
  Mux/1 -> "tout "/1

== system husky_sim_yichu_MPC_test/Controller1/FR  ==
  tgt_angle : Inport
  "current_angle " : Inport  Port=2
  current_omega : Inport  Port=3
  Demux : Demux  Outputs=3
  Demux1 : Demux  Outputs=3
  Demux2 : Demux  Outputs=3
  Mux : Mux  Inputs=3
  "s_joint_ctrl_hip " : Subsystem
  s_joint_ctrl_hip2 : Subsystem
  s_joint_ctrl_knee : Subsystem
  "tout " : Outport
  wires:
  tgt_angle/1 -> Demux/1
  Demux/1 -> "s_joint_ctrl_hip "/1(tgt_angle)
  Demux/2 -> s_joint_ctrl_hip2/1(tgt_angle)
  Demux/3 -> s_joint_ctrl_knee/1(tgt_angle)
  "current_angle "/1 -> Demux1/1
  Demux1/1 -> "s_joint_ctrl_hip "/2("current_angle ")
  Demux1/2 -> s_joint_ctrl_hip2/2("current_angle ")
  Demux1/3 -> s_joint_ctrl_knee/2("current_angle ")
  current_omega/1 -> Demux2/1
  Demux2/1 -> "s_joint_ctrl_hip "/3(current_omega)
  Demux2/2 -> s_joint_ctrl_hip2/3(current_omega)
  Demux2/3 -> s_joint_ctrl_knee/3(current_omega)
  "s_joint_ctrl_hip "/1(tout) -> Mux/1
  s_joint_ctrl_hip2/1(tout) -> Mux/2
  s_joint_ctrl_knee/1(tout) -> Mux/3
  Mux/1 -> "tout "/1

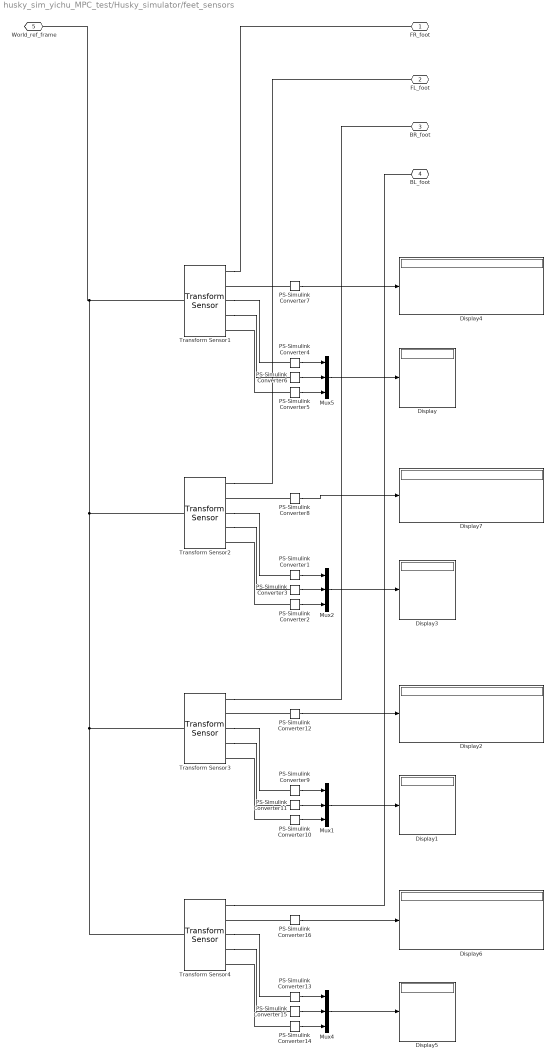
== system husky_sim_yichu_MPC_test/Husky_simulator/feet_sensors ==
  Display{,1..7} (8 alike) : Display
  Mux{1..2,4..5} (4 alike) : Mux  Inputs=3
  PS-Simulink Converter{1..16} (16 alike) : nesl_utility/PS-Simulink Converter  PhysicalDomain=network_engine_domain  SubClassName=ps_output  LeftPortType=input  RightPortType=output  PseudoPeriodic=off  Frequencies=[]  Unit=inherit  AffineConversion=off
  Transform Sensor{1..4} (4 alike) : sm_lib/Frames and Transforms/Transform Sensor  MeasurementFrame=World  SenseAngle=off  SenseAxis=off  SenseAngle1=off  SenseAngle2=off  SenseAngle3=off  SenseQ=off  SenseR=on  SenseOmegaX=off  SenseOmegaY=off  SenseOmegaZ=off  SenseOmega1=off  SenseOmega2=off  SenseOmega3=off  SenseQDot=off  SenseRDot=off  SenseAlphaX=off  SenseAlphaY=off  SenseAlphaZ=off  SenseAlpha1=off  SenseAlpha2=off  SenseAlpha3=off  SenseQDDot=off  SenseRDDot=off  SenseX=on  SenseY=on  SenseZ=on  SenseRad=off  SenseAzim=off  SenseDist=off  SenseInc=off  SenseXDot=off  SenseYDot=off  SenseZDot=off  SenseRadDot=off  SenseAzimDot=off  SenseDistDot=off  SenseIncDot=off  SenseXDDot=off  SenseYDDot=off  SenseZDDot=off  SenseRadDDot=off  SenseAzimDDot=off  SenseDistDDot=off  SenseIncDDot=off
  FR_foot : PMIOPort  Side=Left
  FL_foot : PMIOPort  Port=2  Side=Left
  BR_foot : PMIOPort  Port=3  Side=Left
  BL_foot : PMIOPort  Port=4  Side=Left
  World_ref_frame : PMIOPort  Port=5  Side=Left
  wires:
  Mux5/1 -> Display/1
  PS-Simulink Converter4/1 -> Mux5/1
  PS-Simulink Converter6/1 -> Mux5/2
  PS-Simulink Converter7/1 -> Display4/1
  PS-Simulink Converter5/1 -> Mux5/3
  PS-Simulink Converter14/1 -> Mux4/3
  Mux4/1 -> Display5/1
  PS-Simulink Converter15/1 -> Mux4/2
  PS-Simulink Converter16/1 -> Display6/1
  PS-Simulink Converter13/1 -> Mux4/1
  PS-Simulink Converter10/1 -> Mux1/3
  PS-Simulink Converter9/1 -> Mux1/1
  PS-Simulink Converter12/1 -> Display2/1
  PS-Simulink Converter11/1 -> Mux1/2
  Mux1/1 -> Display1/1
  PS-Simulink Converter2/1 -> Mux2/3
  PS-Simulink Converter1/1 -> Mux2/1
  PS-Simulink Converter8/1 -> Display7/1
  PS-Simulink Converter3/1 -> Mux2/2
  Mux2/1 -> Display3/1
  connections:
  Transform Sensor3/LConn1 -- Transform Sensor4/LConn1 -- Transform Sensor2/LConn1 -- Transform Sensor1/LConn1 -- World_ref_frame/RConn1
  Transform Sensor1/RConn1 -- FR_foot/RConn1
  Transform Sensor3/RConn1 -- BR_foot/RConn1
  Transform Sensor4/RConn1 -- BL_foot/RConn1
  Transform Sensor2/RConn1 -- FL_foot/RConn1
  Transform Sensor4/RConn4 -- PS-Simulink Converter15/LConn1
  PS-Simulink Converter12/LConn1 -- Transform Sensor3/RConn2
  Transform Sensor3/RConn3 -- PS-Simulink Converter9/LConn1
  Transform Sensor4/RConn3 -- PS-Simulink Converter13/LConn1
  Transform Sensor3/RConn4 -- PS-Simulink Converter11/LConn1
  PS-Simulink Converter7/LConn1 -- Transform Sensor1/RConn2
  Transform Sensor2/RConn4 -- PS-Simulink Converter3/LConn1
  Transform Sensor1/RConn4 -- PS-Simulink Converter6/LConn1
  PS-Simulink Converter10/LConn1 -- Transform Sensor3/RConn5
  PS-Simulink Converter5/LConn1 -- Transform Sensor1/RConn5
  Transform Sensor2/RConn3 -- PS-Simulink Converter1/LConn1
  PS-Simulink Converter8/LConn1 -- Transform Sensor2/RConn2
  PS-Simulink Converter16/LConn1 -- Transform Sensor4/RConn2
  PS-Simulink Converter14/LConn1 -- Transform Sensor4/RConn5
  PS-Simulink Converter2/LConn1 -- Transform Sensor2/RConn5
  Transform Sensor1/RConn3 -- PS-Simulink Converter4/LConn1

== system husky_sim_yichu_MPC_test/Husky_simulator/foot end from FK  ==
  sensor_input_angles : Inport
  MATLAB Function : MATLAB Function  TreatAsAtomicUnit=on
  "foot_end_position " : Outport
  wires:
  sensor_input_angles/1 -> MATLAB Function/1(sensor_input)
  MATLAB Function/1(foot_end_position) -> "foot_end_position "/1

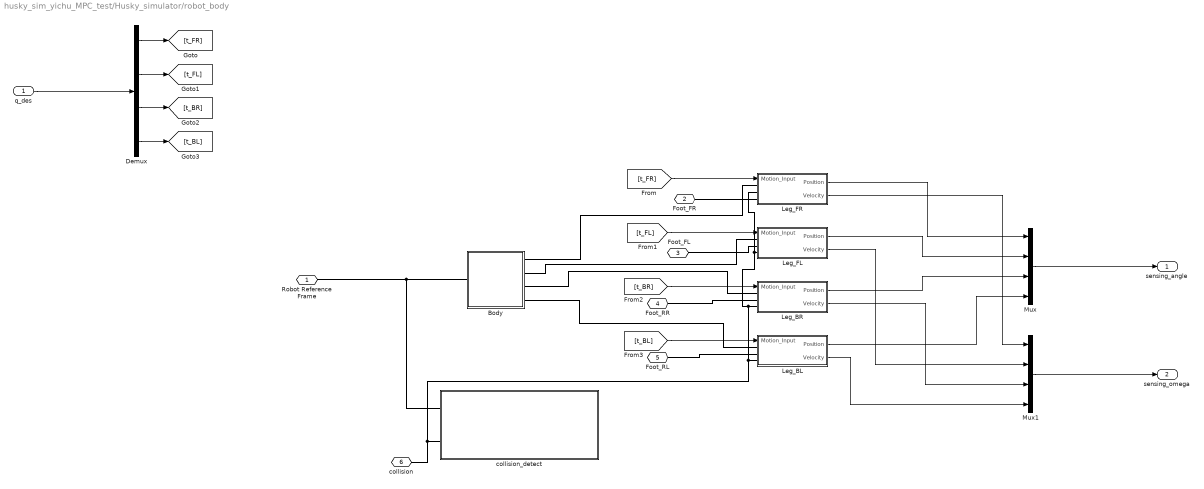
== system husky_sim_yichu_MPC_test/Husky_simulator/robot_body ==
  q_des : Inport
  Body : Subsystem
  Demux : Demux
  Leg_BL : Subsystem
  Leg_BR : Subsystem
  Leg_FL : Subsystem
  Leg_FR : Subsystem
  Mux : Mux
  Mux1 : Mux
  "collision_detect " : Subsystem
  Robot Reference Frame : PMIOPort  Side=Left
  Foot_FR : PMIOPort  Port=2  Side=Left
  Foot_FL : PMIOPort  Port=3  Side=Left
  Foot_RR : PMIOPort  Port=4  Side=Left
  Foot_RL : PMIOPort  Port=5  Side=Left
  "collision " : PMIOPort  Port=6  Side=Left
  sensing_angle : Outport  VectorParamsAs1DForOutWhenUnconnected=off
  sensing_omega : Outport  Port=2  VectorParamsAs1DForOutWhenUnconnected=off
  wires:
  q_des/1 -> Demux/1
  Demux/1 -> [t_FR]
  Demux/2 -> [t_FL]
  Demux/3 -> [t_BR]
  Demux/4 -> [t_BL]
  Mux/1 -> sensing_angle/1
  Leg_FR/1(Position) -> Mux/1
  [t_FR] -> Leg_FR/1(Motion_Input)
  Leg_BR/1(Position) -> Mux/3
  [t_FL] -> Leg_FL/1(Motion_Input)
  [t_BR] -> Leg_BR/1(Motion_Input)
  Leg_FL/1(Position) -> Mux/2
  Leg_BL/1(Position) -> Mux/4
  [t_BL] -> Leg_BL/1(Motion_Input)
  Leg_FL/2(Velocity) -> Mux1/2
  Leg_BR/2(Velocity) -> Mux1/3
  Leg_BL/2(Velocity) -> Mux1/4
  Leg_FR/2(Velocity) -> Mux1/1
  Mux1/1 -> sensing_omega/1
  connections:
  Body/LConn1 -- "collision_detect "/LConn1 -- Robot Reference Frame/RConn1
  Body/RConn1 -- Leg_FR/LConn1
  Foot_FR/RConn1 -- Leg_FR/LConn2
  Body/RConn2 -- Leg_FL/LConn1
  Foot_RL/RConn1 -- Leg_BL/LConn2
  Leg_BR/LConn2 -- Foot_RR/RConn1
  Body/RConn3 -- Leg_BR/LConn1
  Body/RConn4 -- Leg_BL/LConn1
  Foot_FL/RConn1 -- Leg_FL/LConn2
  Leg_FR/LConn3 -- "collision "/RConn1 -- "collision_detect "/LConn2 -- Leg_BL/LConn3 -- Leg_BR/LConn3 -- Leg_FL/LConn3

== system husky_sim_yichu_MPC_test/Husky_simulator/visualize position in space  ==
  position input : Inport
  Demux : Demux
  Scope : Scope
  Subsystem : Subsystem
  Subsystem1 : Subsystem
  Subsystem2 : Subsystem
  Subsystem4 : Subsystem
  robot reference : PMIOPort  Tag=PMCPort  Side=Left
  wires:
  position input/1 -> Scope/1, Demux/1
  Demux/1 -> Subsystem/1(In1)
  Demux/2 -> Subsystem4/1(In1)
  Demux/3 -> Subsystem1/1(In1)
  Demux/4 -> Subsystem2/1(In1)
  connections:
  Subsystem2/LConn1 -- robot reference/RConn1 -- Subsystem1/LConn1 -- Subsystem4/LConn1 -- Subsystem/LConn1

== system husky_sim_yichu_MPC_test/Controller/BL/s_joint_ctrl_hip  ==
  tgt_angle : Inport
  "current_angle " : Inport  Port=2
  current_omega : Inport  Port=3
  PID Controller : simulink/Continuous/PID Controller  Controller=PID  Form=Parallel  TimeDomain=Continuous-time  SampleTime=-1  IntegratorMethod=Forward Euler  FilterMethod=Forward Euler  ControllerParametersSource=internal  P=hipf_ctrl.pos_kp  I=hipf_ctrl.pos_ki  D=hipf_ctrl.pos_kd  UseFilter=on  N=100  TunerSelectOption=Transfer Function Based (PID Tuner App)  InitialConditionSource=internal  InitialConditionForIntegrator=0  InitialConditionForFilter=0  DifferentiatorICPrevScaledInput=0  ExternalReset=none  TrackingMode=off  Kt=1  LimitOutput=off  UpperSaturationLimit=inf  LowerSaturationLimit=-inf  LinearizeAsGain=on  AntiWindupMode=none  Kb=1  POutMin=[]  POutMax=[]  IOutMin=[]  IOutMax=[]  DOutMin=[]  DOutMax=[]  NOutMin=[]  NOutMax=[]  SumOutMin=[]  SumOutMax=[]  SaturationOutMin=[]  SaturationOutMax=[]  PParamMin=[]  PParamMax=[]  IParamMin=[]  IParamMax=[]  DParamMin=[]  DParamMax=[]  NParamMin=[]  NParamMax=[]  KbParamMin=[]  KbParamMax=[]  KtParamMin=[]  KtParamMax=[]  KbOutMin=[]  KbOutMax=[]  KtOutMin=[]  KtOutMax=[]  IntegratorOutMin=[]  IntegratorOutMax=[]  FilterOutMin=[]  FilterOutMax=[]  SumI1OutMin=[]  SumI1OutMax=[]  SumI2OutMin=[]  SumI2OutMax=[]  SumI3OutMin=[]  SumI3OutMax=[]  SumI4OutMin=[]  SumI4OutMax=[]  SumDOutMin=[]  SumDOutMax=[]  DifferentiatorOutMin=[]  DifferentiatorOutMax=[]  FilterDiffOutCoefMin=[]  FilterDiffOutCoefMax=[]  ReciprocalOutMin=[]  ReciprocalOutMax=[]  SumDenOutMin=[]  SumDenOutMax=[]  SumNumOutMin=[]  SumNumOutMax=[]  DivideOutMin=[]  DivideOutMax=[]  IntegratorContinuousStateAttributes=''  IntegratorStateMustResolveToSignalObject=off  IntegratorRTWStateStorageClass=Auto  FilterContinuousStateAttributes=''  FilterStateMustResolveToSignalObject=off  FilterRTWStateStorageClass=Auto  ParallelPVariant=InternalParameters  IdealPVariant=Disabled  IVariant=InternalParameters  DVariant=InternalParameters  IntegratorVariant=Continuous  SatVariant=Disabled  AWVariant=Passthrough  PCopyVariant=Disabled  TRVariant=Disabled  FdbkBlocksVariant=Forward  IdealPFdbkVariant=Disabled  SatFdbkVariant=Disabled  DerivativeFilterVariant=ContFilter  NVariant=InternalParameters  NCopyVariant=Disabled  FilterICVariant=InternalICsFilter  IntegratorICVariant=InternalICs  ExternalResetVariant=Disabled  TRSumVariant=Passthrough  SumFdbkVariant=Disabled  SumVariant=Sum_PID
  PID Controller3 : simulink/Continuous/PID Controller  Controller=PID  Form=Parallel  TimeDomain=Continuous-time  SampleTime=-1  IntegratorMethod=Forward Euler  FilterMethod=Forward Euler  ControllerParametersSource=internal  P=hipf_ctrl.vel_kp  I=hipf_ctrl.vel_ki  D=hipf_ctrl.vel_kd  UseFilter=on  N=100  TunerSelectOption=Transfer Function Based (PID Tuner App)  InitialConditionSource=internal  InitialConditionForIntegrator=0  InitialConditionForFilter=0  DifferentiatorICPrevScaledInput=0  ExternalReset=none  TrackingMode=off  Kt=1  LimitOutput=off  UpperSaturationLimit=inf  LowerSaturationLimit=-inf  LinearizeAsGain=on  AntiWindupMode=none  Kb=1  POutMin=[]  POutMax=[]  IOutMin=[]  IOutMax=[]  DOutMin=[]  DOutMax=[]  NOutMin=[]  NOutMax=[]  SumOutMin=[]  SumOutMax=[]  SaturationOutMin=[]  SaturationOutMax=[]  PParamMin=[]  PParamMax=[]  IParamMin=[]  IParamMax=[]  DParamMin=[]  DParamMax=[]  NParamMin=[]  NParamMax=[]  KbParamMin=[]  KbParamMax=[]  KtParamMin=[]  KtParamMax=[]  KbOutMin=[]  KbOutMax=[]  KtOutMin=[]  KtOutMax=[]  IntegratorOutMin=[]  IntegratorOutMax=[]  FilterOutMin=[]  FilterOutMax=[]  SumI1OutMin=[]  SumI1OutMax=[]  SumI2OutMin=[]  SumI2OutMax=[]  SumI3OutMin=[]  SumI3OutMax=[]  SumI4OutMin=[]  SumI4OutMax=[]  SumDOutMin=[]  SumDOutMax=[]  DifferentiatorOutMin=[]  DifferentiatorOutMax=[]  FilterDiffOutCoefMin=[]  FilterDiffOutCoefMax=[]  ReciprocalOutMin=[]  ReciprocalOutMax=[]  SumDenOutMin=[]  SumDenOutMax=[]  SumNumOutMin=[]  SumNumOutMax=[]  DivideOutMin=[]  DivideOutMax=[]  IntegratorContinuousStateAttributes=''  IntegratorStateMustResolveToSignalObject=off  IntegratorRTWStateStorageClass=Auto  FilterContinuousStateAttributes=''  FilterStateMustResolveToSignalObject=off  FilterRTWStateStorageClass=Auto  ParallelPVariant=InternalParameters  IdealPVariant=Disabled  IVariant=InternalParameters  DVariant=InternalParameters  IntegratorVariant=Continuous  SatVariant=Disabled  AWVariant=Passthrough  PCopyVariant=Disabled  TRVariant=Disabled  FdbkBlocksVariant=Forward  IdealPFdbkVariant=Disabled  SatFdbkVariant=Disabled  DerivativeFilterVariant=ContFilter  NVariant=InternalParameters  NCopyVariant=Disabled  FilterICVariant=InternalICsFilter  IntegratorICVariant=InternalICs  ExternalResetVariant=Disabled  TRSumVariant=Passthrough  SumFdbkVariant=Disabled  SumVariant=Sum_PID
  Sum1 : Sum  Inputs=|+-
  Sum6 : Sum  Inputs=|+-
  tout : Outport
  wires:
  current_omega/1 -> Sum6/2
  "current_angle "/1 -> Sum1/2
  Sum6/1 -> PID Controller3/1
  PID Controller/1 -> Sum6/1
  Sum1/1 -> PID Controller/1
  tgt_angle/1 -> Sum1/1
  PID Controller3/1 -> tout/1
